simulink model "ecelp_sq"  (Simulink 6.1)
settings: Solver=FixedStepDiscrete  SolverMode=SingleTasking  StartTime=0.0  StopTime=3  RelTol=1e-3
PreLoadFcn:
  | load lpcvocoder.mat;
undefined symbols (not defined in the file): magnitude, poly2lsf
libraries: simulink x26, dspquant2 x26, dspindex x18, dspcelplib x14, dsparch4 x12, dspstat3 x10, dspsrcs4 x9, dspsigops x7, dsplp x5, dspmtrx3 x3, dspbuff3 x2, dspsolvers x1
(part 4 of 4)

== system ecelp_sq/CELP Encoder/Frame Analysis/LSF Vector Quantization/LSF xQ./for6to10/Subsystem3 ==
  lsf_i : Inport  Port=1  LatchInput=off
  SQ Decoder : dspquant2/Scalar Quantizer Decoder  Tag=SQDESIGN_GUI_REALIZE_MODEL  CBsource=Specify via dialog  invalidin=Clip  codebook=finalCB9  dataType=double  isSigned=on  wordLen=16  udDataType=sfix(16)  fracBitsMode=Best precision  numFracBits=11
  SQ Encoder : dspquant2/Scalar Quantizer Encoder  Tag=SQDESIGN_GUI_REALIZE_MODEL  paramSrc=Specify via dialog  partType=Bounded  BBoundary=finalBP9  UBoundary="[ 0.099974     0.10302     0.10488     0.10701     0.10913     0.11147     0.11383     0.11573     0.11716     0.11878      0.1209     0.12301     0.12507     0.12713     0.12913     0.13116     0.13321     0.13537     0.13749     0.13936     0.14111     0.14279     0.14444     0.14618     0.14802     0.14992     0.15185     0.15381     0.15583      0.1579     0.15992     0.16188     0.16386     0.16587     0.16795      0.1702     0.17247      0.1746     0.17673     0.17871     0.18049     0.18224     0.18415     0.18623     0.18831     0.19034     0.19244     0.19453     0.19655     0.19854     0.20052     0.20252     0.20456     0.20661     0.20877     0.21096     0.21304     0.21507     0.21708     0.21911     0.22111     0.22317     0.22525     0.22727     0.22926     0.23137     0.23346     0.23545     0.23752      0.2396     0.24154     0.24351     0.24557     0.24763     0.24971     0.25186     0.25395      0.2559     0.25777     0.25964     0.26159     0.26362     0.26562     0.26763     0.26971     0.27179     0.27389     0.27604     0.27823     0.28043     0.28249     0.28434     0.28604     0.28793     0.29009      0.2923     0.29456     0.29667     0.29862     0.30064     0.30262     0.30452     0.30638     0.30839     0.31058     0.31276     0.31497     0.31719      0.3191     0.32081     0.32252     0.32426     0.32606     0.32766     0.32935     0.33118     0.33302      0.3346     0.33596     0.33751     0.33902     0.34044      0.3419     0.34326     0.34442     0.34549      0.3465     0.34753     0.34856     0.34955     0.35043     0.35125     0.35211     0.35301     0.35391     0.35469     0.35547     0.35637     0.35724     0.35811       0.359     0.35976     0.36034     0.36104     0.36191     0.36281     0.36378     0.36468     0.36553     0.36633     0.36703     0.36774      0.3685     0.36932     0.37019     0.37095     0.37175     0.37258     0.37334     0.37423     0.37503     0.37578     0.37649     0.37709     0.37779      0.3785     0.37908     0.37979     0.38066     0.38144     0.38216     0.38292     0.38373     0.38449     0.38515     0.38587      0.3866     0.38739      0.3881     0.38859     0.38929     0.39005     0.39064     0.39142     0.39247     0.39343      0.3942     0.39484      0.3954     0.39609     0.39678     0.39739     0.39826     0.39943     0.40069     0.40224     0.40416     0.40656     0.40863     0.41013     0.41235     0.41481     0.41687     0.41887     0.42088     0.42275     0.42476     0.42715     0.42951     0.43142     0.43308     0.43504     0.43726      0.4392     0.44117      0.4432     0.44511       0.447      0.4491     0.45098     0.45311     0.45561     0.45757     0.45946     0.46152     0.46332     0.46532     0.46772     0.46983     0.47269     0.47636     0.47892      0.4802     0.48193     0.48413     0.48628     0.48855     0.49142     0.49443     0.49619     0.49825     0.50069     0.50458     0.50844      0.5118     0.51615      0.5214     0.52728     0.53525     0.54339      0.5515     0.56113     0.57486     0.59255     0.60963  ]"  SearchMethod=Binary  tieBreakRule=Choose the lower index  outQU=off  outQError=off  codebook="[0.097671     0.10228     0.10377       0.106     0.10803     0.11023     0.11271     0.11496     0.11651     0.11781     0.11975     0.12206     0.12397     0.12616      0.1281     0.13016     0.13216     0.13426     0.13648     0.13849     0.14023     0.14199      0.1436     0.14527     0.14709     0.14895      0.1509     0.15281     0.15481     0.15685     0.15895     0.16088     0.16288     0.16484      0.1669     0.16901      0.1714     0.17354     0.17567     0.17778     0.17963     0.18136     0.18313     0.18517     0.18729     0.18933     0.19135     0.19353     0.19553     0.19757     0.19952     0.20152     0.20351     0.20561     0.20762     0.20992     0.21199     0.21409     0.21605     0.21811      0.2201     0.22211     0.22422     0.22628     0.22825     0.23027     0.23247     0.23446     0.23644      0.2386     0.24059     0.24248     0.24454      0.2466     0.24865     0.25077     0.25295     0.25494     0.25687     0.25868     0.26059     0.26259     0.26464      0.2666     0.26865     0.27076     0.27282     0.27496     0.27712     0.27934     0.28151     0.28348     0.28521     0.28687     0.28898     0.29119      0.2934     0.29571     0.29763     0.29962     0.30166     0.30358     0.30546      0.3073     0.30947     0.31168     0.31383     0.31611     0.31826     0.31993     0.32168     0.32335     0.32517     0.32694     0.32838     0.33031     0.33204     0.33401      0.3352     0.33673     0.33829     0.33976     0.34112     0.34268     0.34384     0.34499     0.34599     0.34701     0.34804     0.34907     0.35004     0.35083     0.35167     0.35255     0.35346     0.35436     0.35503     0.35591     0.35682     0.35765     0.35856     0.35944     0.36007     0.36061     0.36148     0.36233     0.36329     0.36427     0.36508     0.36598     0.36667     0.36738     0.36811     0.36889     0.36975     0.37064     0.37127     0.37223     0.37293     0.37375     0.37471     0.37534     0.37622     0.37677      0.3774     0.37817     0.37882     0.37934     0.38023      0.3811     0.38178     0.38254      0.3833     0.38416     0.38482     0.38549     0.38625     0.38695     0.38783     0.38838     0.38881     0.38976     0.39034     0.39094      0.3919     0.39304     0.39383     0.39458      0.3951     0.39571     0.39646      0.3971     0.39769     0.39884     0.40003     0.40135     0.40314     0.40519     0.40794     0.40932     0.41094     0.41375     0.41586     0.41787     0.41988     0.42187     0.42362     0.42589     0.42841     0.43061     0.43222     0.43394     0.43615     0.43836     0.44004     0.44231     0.44409     0.44613     0.44787     0.45033     0.45164     0.45459     0.45664      0.4585     0.46042     0.46262     0.46401     0.46663     0.46882     0.47084     0.47455     0.47818     0.47966     0.48075     0.48312     0.48514     0.48742     0.48968     0.49315     0.49571     0.49666     0.49984     0.50154     0.50761     0.50927     0.51434     0.51795     0.52484     0.52971     0.54078     0.54599     0.55701     0.56525     0.58448     0.60063     0.61863]"  outStatus=off  invalidin=Clip  idtype=int32  roundingMode=Floor  overflowMode=off
  ind_i : Outport
  ulsf_i : Outport  Port=2
  wires:
  SQ Encoder/1 -> SQ Decoder/1, ind_i/1
  lsf_i/1 -> SQ Encoder/1
  SQ Decoder/1 -> ulsf_i/1

== system ecelp_sq/CELP Encoder/Frame Analysis/LSF Vector Quantization/LSF xQ./for6to10/Subsystem4 ==
  lsf_i : Inport  Port=1  LatchInput=off
  SQ Decoder : dspquant2/Scalar Quantizer Decoder  Tag=SQDESIGN_GUI_REALIZE_MODEL  CBsource=Specify via dialog  invalidin=Clip  codebook=finalCB10  dataType=double  isSigned=on  wordLen=16  udDataType=sfix(16)  fracBitsMode=Best precision  numFracBits=11
  SQ Encoder : dspquant2/Scalar Quantizer Encoder  Tag=SQDESIGN_GUI_REALIZE_MODEL  paramSrc=Specify via dialog  partType=Bounded  BBoundary=finalBP10  UBoundary="[ 0.099974     0.10302     0.10488     0.10701     0.10913     0.11147     0.11383     0.11573     0.11716     0.11878      0.1209     0.12301     0.12507     0.12713     0.12913     0.13116     0.13321     0.13537     0.13749     0.13936     0.14111     0.14279     0.14444     0.14618     0.14802     0.14992     0.15185     0.15381     0.15583      0.1579     0.15992     0.16188     0.16386     0.16587     0.16795      0.1702     0.17247      0.1746     0.17673     0.17871     0.18049     0.18224     0.18415     0.18623     0.18831     0.19034     0.19244     0.19453     0.19655     0.19854     0.20052     0.20252     0.20456     0.20661     0.20877     0.21096     0.21304     0.21507     0.21708     0.21911     0.22111     0.22317     0.22525     0.22727     0.22926     0.23137     0.23346     0.23545     0.23752      0.2396     0.24154     0.24351     0.24557     0.24763     0.24971     0.25186     0.25395      0.2559     0.25777     0.25964     0.26159     0.26362     0.26562     0.26763     0.26971     0.27179     0.27389     0.27604     0.27823     0.28043     0.28249     0.28434     0.28604     0.28793     0.29009      0.2923     0.29456     0.29667     0.29862     0.30064     0.30262     0.30452     0.30638     0.30839     0.31058     0.31276     0.31497     0.31719      0.3191     0.32081     0.32252     0.32426     0.32606     0.32766     0.32935     0.33118     0.33302      0.3346     0.33596     0.33751     0.33902     0.34044      0.3419     0.34326     0.34442     0.34549      0.3465     0.34753     0.34856     0.34955     0.35043     0.35125     0.35211     0.35301     0.35391     0.35469     0.35547     0.35637     0.35724     0.35811       0.359     0.35976     0.36034     0.36104     0.36191     0.36281     0.36378     0.36468     0.36553     0.36633     0.36703     0.36774      0.3685     0.36932     0.37019     0.37095     0.37175     0.37258     0.37334     0.37423     0.37503     0.37578     0.37649     0.37709     0.37779      0.3785     0.37908     0.37979     0.38066     0.38144     0.38216     0.38292     0.38373     0.38449     0.38515     0.38587      0.3866     0.38739      0.3881     0.38859     0.38929     0.39005     0.39064     0.39142     0.39247     0.39343      0.3942     0.39484      0.3954     0.39609     0.39678     0.39739     0.39826     0.39943     0.40069     0.40224     0.40416     0.40656     0.40863     0.41013     0.41235     0.41481     0.41687     0.41887     0.42088     0.42275     0.42476     0.42715     0.42951     0.43142     0.43308     0.43504     0.43726      0.4392     0.44117      0.4432     0.44511       0.447      0.4491     0.45098     0.45311     0.45561     0.45757     0.45946     0.46152     0.46332     0.46532     0.46772     0.46983     0.47269     0.47636     0.47892      0.4802     0.48193     0.48413     0.48628     0.48855     0.49142     0.49443     0.49619     0.49825     0.50069     0.50458     0.50844      0.5118     0.51615      0.5214     0.52728     0.53525     0.54339      0.5515     0.56113     0.57486     0.59255     0.60963  ]"  SearchMethod=Binary  tieBreakRule=Choose the lower index  outQU=off  outQError=off  codebook="[0.097671     0.10228     0.10377       0.106     0.10803     0.11023     0.11271     0.11496     0.11651     0.11781     0.11975     0.12206     0.12397     0.12616      0.1281     0.13016     0.13216     0.13426     0.13648     0.13849     0.14023     0.14199      0.1436     0.14527     0.14709     0.14895      0.1509     0.15281     0.15481     0.15685     0.15895     0.16088     0.16288     0.16484      0.1669     0.16901      0.1714     0.17354     0.17567     0.17778     0.17963     0.18136     0.18313     0.18517     0.18729     0.18933     0.19135     0.19353     0.19553     0.19757     0.19952     0.20152     0.20351     0.20561     0.20762     0.20992     0.21199     0.21409     0.21605     0.21811      0.2201     0.22211     0.22422     0.22628     0.22825     0.23027     0.23247     0.23446     0.23644      0.2386     0.24059     0.24248     0.24454      0.2466     0.24865     0.25077     0.25295     0.25494     0.25687     0.25868     0.26059     0.26259     0.26464      0.2666     0.26865     0.27076     0.27282     0.27496     0.27712     0.27934     0.28151     0.28348     0.28521     0.28687     0.28898     0.29119      0.2934     0.29571     0.29763     0.29962     0.30166     0.30358     0.30546      0.3073     0.30947     0.31168     0.31383     0.31611     0.31826     0.31993     0.32168     0.32335     0.32517     0.32694     0.32838     0.33031     0.33204     0.33401      0.3352     0.33673     0.33829     0.33976     0.34112     0.34268     0.34384     0.34499     0.34599     0.34701     0.34804     0.34907     0.35004     0.35083     0.35167     0.35255     0.35346     0.35436     0.35503     0.35591     0.35682     0.35765     0.35856     0.35944     0.36007     0.36061     0.36148     0.36233     0.36329     0.36427     0.36508     0.36598     0.36667     0.36738     0.36811     0.36889     0.36975     0.37064     0.37127     0.37223     0.37293     0.37375     0.37471     0.37534     0.37622     0.37677      0.3774     0.37817     0.37882     0.37934     0.38023      0.3811     0.38178     0.38254      0.3833     0.38416     0.38482     0.38549     0.38625     0.38695     0.38783     0.38838     0.38881     0.38976     0.39034     0.39094      0.3919     0.39304     0.39383     0.39458      0.3951     0.39571     0.39646      0.3971     0.39769     0.39884     0.40003     0.40135     0.40314     0.40519     0.40794     0.40932     0.41094     0.41375     0.41586     0.41787     0.41988     0.42187     0.42362     0.42589     0.42841     0.43061     0.43222     0.43394     0.43615     0.43836     0.44004     0.44231     0.44409     0.44613     0.44787     0.45033     0.45164     0.45459     0.45664      0.4585     0.46042     0.46262     0.46401     0.46663     0.46882     0.47084     0.47455     0.47818     0.47966     0.48075     0.48312     0.48514     0.48742     0.48968     0.49315     0.49571     0.49666     0.49984     0.50154     0.50761     0.50927     0.51434     0.51795     0.52484     0.52971     0.54078     0.54599     0.55701     0.56525     0.58448     0.60063     0.61863]"  outStatus=off  invalidin=Clip  idtype=int32  roundingMode=Floor  overflowMode=off
  ind_i : Outport
  ulsf_i : Outport  Port=2
  wires:
  SQ Encoder/1 -> SQ Decoder/1, ind_i/1
  lsf_i/1 -> SQ Encoder/1
  SQ Decoder/1 -> ulsf_i/1

== system ecelp_sq/CELP Encoder/Subframe Analysis/Innovation signal quantization/Searching for FCB pulse  positions and FCB gain/Optimal Features/Local maxima detector ==
  note: Note: The 'Running Maximum' block
      | exploits the reset option in 'For' iterator
  Err : Inport  Port=1  LatchInput=off
  Relational Operator1 : RelationalOperator  Operator===  LogicOutDataTypeMode=Boolean  InputSameDT=on
  Running Maximum : dspstat3/Maximum  DialogController=dspDDGCreate  DialogControllerArgs=DataTag19  fcn=Running  reset=None  roundingMode=Floor  overflowMode=off
  Flag : Outport
  wires:
  Err/1 -> Running Maximum/1, Relational Operator1/1
  Running Maximum/1 -> Relational Operator1/2
  Relational Operator1/1 -> Flag/1
